simulink model "boost_converter_frequency_response"  (R2024b)
settings: Solver=ode3  StartTime=0.0  StopTime=10  RelTol=1e-3  EnableMultiTasking=on
libraries: arduinolib x2
settings Model: SimulationMode=external  ExtModeTrigDuration=2  Creator=gcampa  LastModifiedBy=Anhad Mehrotra
settings SolverCC: AlgebraicLoopSolver=TrustRegion  AutoInsertRateTranBlk=on
settings DataIOCC: LimitDataPoints=on  SaveFormat=Array  ReturnWorkspaceOutputs=off
settings OptimizationCC: EnhancedBackFolding=on  PassReuseOutputArgsAs=Individual arguments  ZeroExternalMemoryAtStartup=off  ZeroInternalMemoryAtStartup=off  MaxStackSize=64  OptimizeBlockOrder=speed  DifferentSizesBufferReuse=on  OptimizationCustomize=off  EfficientTunableParamExpr=on
settings DebuggingCC: UnderspecifiedInitializationDetection=Classic  MergeDetectMultiDrivingBlocksExec=none  ParameterTunabilityLossMsg=error  UnconnectedInputMsg=warning  UnconnectedOutputMsg=warning  UnconnectedLineMsg=warning  SFUnexpectedBacktrackingDiag=warning  SFNoUnconditionalDefaultTransitionDiag=warning  SFExecutionAtInitializationDiag=none  ArithmeticOperatorsInVariantConditions=warning
settings HardwareCC: ProdBitPerInt=16  ProdBitPerPointer=16  ProdBitPerSizeT=16  ProdBitPerPtrDiffT=16  ProdLargestAtomicFloat=None  ProdWordSize=8  ProdHWDeviceType=Atmel->AVR  UseEmbeddedCoderFeatures=off  UseSimulinkCoderFeatures=off
settings ModelReferenceCC: PropagateSignalLabelsOutOfModel=off
settings SFSimCC: SimUseLocalCustomCode=off  MATLABDynamicMemAlloc=off  CustomCodeUndefinedFunction=UseInterfaceOnly
settings RTWCC: Description=Embedded Coder  SystemTargetFile=ert.tlc  HardwareBoard=Arduino Uno  TemplateMakefile=ert_default_tmf  RTWVerbose=off  RTWUseLocalCustomCode=off  Toolchain=Arduino AVR  BuildConfiguration=Faster Runs  GPUComputeCapability=3.5
settings CodeAppCC: ForceParamTrailComments=on  IgnoreCustomStorageClasses=off  OperatorAnnotations=on  SimulinkDataObjDesc=on  SFDataObjDesc=on  InsertBlockDesc=on
settings ERTTargetCC: SupportContinuousTime=on  SupportNonInlinedSFcns=on  SupportVariableSizeSignals=on  ExtModeTransport=3  ExtModeStaticAlloc=on  ExtModeAutomaticAllocSize=off  ExtModeStaticAllocSize=250  ExtModeMexFile=ext_xcp  ExtModeIntrfLevel=Level2 - Open  InlinedParameterPlacement=Hierarchical
settings ConfigComp: CovMetricSettings=dw  CovSaveCumulativeToWorkspaceVar=on  CovSaveSingleToWorkspaceVar=on  CovExternalEMLEnable=off

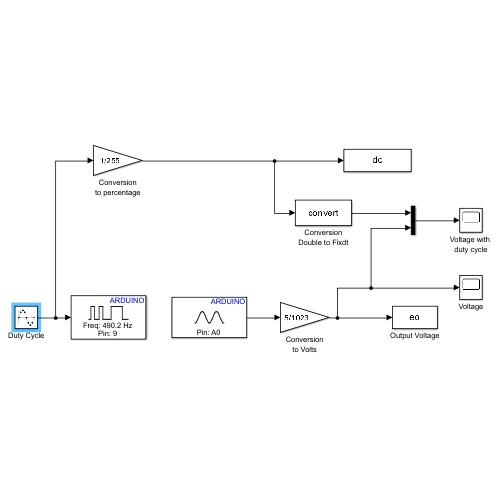
[thumbnail: Simulink's stored preview of the top-level diagram]
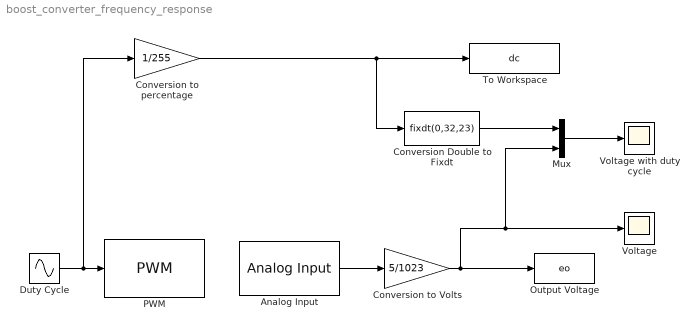
== system boost_converter_frequency_response ==
  Analog Input : arduinolib/Analog Input  pinNumber=0  ReadResultsOnly=off  ConversionTriggerSource=Software  ExternalTriggerType=uint32( 0 )  OutputDataType=uint16  EnableConversionCompleteNotify=off  EnableOuputStatus=off  SampleTime=-1  blockPlatform=arduino
  Conversion Double to Fixdt : DataTypeConversion  OutDataTypeStr=fixdt(0,32,23)  SaturateOnIntegerOverflow=off  RndMeth=Floor
  Conversion to Volts : Gain  Gain=5/1023
  Conversion to percentage : Gain  Gain=1/255
  Duty Cycle : Sin  SineType=Sample based  Amplitude=40  Bias=100  Frequency=10*pi  SampleTime=0.01  Offset=1*pi
  Mux : Mux  Inputs=2
  Output Voltage : ToWorkspace  VariableName=eo  SampleTime=-1
      settings: Save2DSignal=2-D array (concatenate along first dimension)
  PWM : arduinolib/PWM  pinNumber=9  frequencyType=Specify  desiredFrequency=490.2  achievableFrequency=490.1961
  To Workspace : ToWorkspace  VariableName=dc  SampleTime=-1
      settings: Save2DSignal=2-D array (concatenate along first dimension)
  Voltage : Scope
  Voltage with duty cycle : Scope
  wires:
  Analog Input/1 -> Conversion to Volts/1
  Conversion to Volts/1 -> Mux/2, Voltage/1, Output Voltage/1
  Conversion to percentage/1 -> Conversion Double to Fixdt/1, To Workspace/1
  Duty Cycle/1 -> PWM/1, Conversion to percentage/1
  Conversion Double to Fixdt/1 -> Mux/1
  Mux/1 -> Voltage with duty cycle/1
